simulink model "robot"  (R2019b)
settings: Solver=VariableStepAuto  StartTime=0.0  StopTime=45  RelTol=1e-3
values from neighbouring files (symbols this model uses):
  kf = 20    [workspace.mat]
  km = 0.4872    [workspace.mat]
  kp = 10    [workspace.mat]
  momemt_of_inertia = 0.0024    [workspace.mat]
  targets = [1  1; 2  1; -1  -1; -1  1; 0  0]    [workspace.mat]
  wheel_radius = 0.02    [workspace.mat]
  wheel_span = 0.1    [workspace.mat]
  winding_inductance = 0.0047    [workspace.mat]
  winding_resistance = 8.4929    [workspace.mat]
libraries: dspsigops x1, simulink x1
settings Model: Creator=Gudini  LastModifiedBy=Gudini

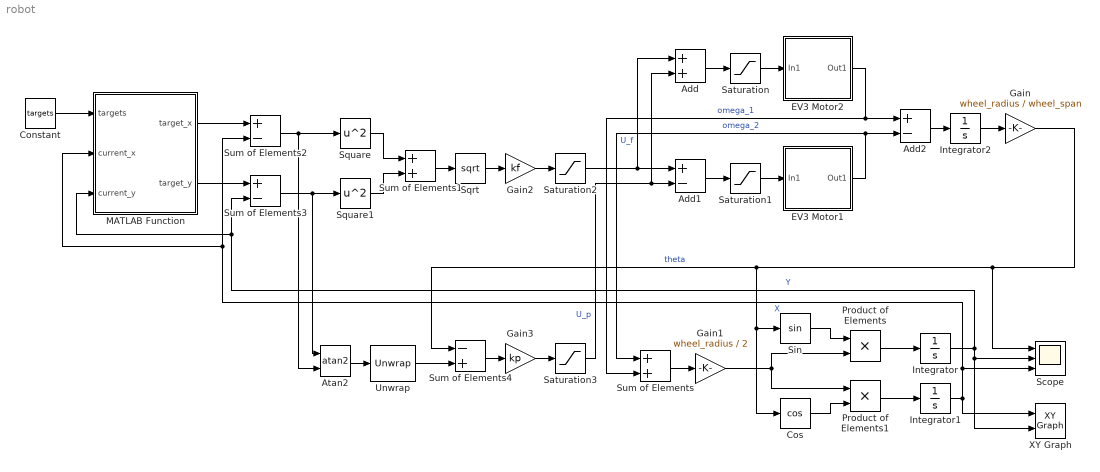
== system robot ==
  Add : Sum
  Add1 : Sum  Inputs=+-
  Add2 : Sum  Inputs=+-
  Atan2 : Trigonometry  Operator=atan2
  Constant : Constant  Value=targets  VectorParams1D=off
  Cos : Trigonometry  Operator=cos
  EV3 Motor1 : Subsystem
  EV3 Motor2 : Subsystem
  Gain : Gain  Gain=wheel_radius / wheel_span
  Gain1 : Gain  Gain=wheel_radius / 2
  Gain2 : Gain  Gain=kf
  Gain3 : Gain  Gain=kp
  Integrator : Integrator
  Integrator1 : Integrator
  Integrator2 : Integrator
  MATLAB Function : MATLAB Function  TreatAsAtomicUnit=on
  Product of Elements : Product
  Product of Elements1 : Product
  Saturation : Saturate  UpperLimit=7.6  LowerLimit=-7.6  ZeroCross=off
  Saturation1 : Saturate  UpperLimit=7.6  LowerLimit=-7.6  ZeroCross=off
  Saturation2 : Saturate  UpperLimit=7.6  LowerLimit=-7.6
  Saturation3 : Saturate  UpperLimit=7.6  LowerLimit=-7.6
  Scope : Scope  NumInputPorts=3
  Sin : Trigonometry
  Sqrt : Sqrt  SaturateOnIntegerOverflow=on
  Square : Math  Operator=square  SignedPower=off  SaturateOnIntegerOverflow=on
  Square1 : Math  Operator=square  SignedPower=off  SaturateOnIntegerOverflow=on
  Sum of Elements : Sum
  Sum of Elements1 : Sum
  Sum of Elements2 : Sum  Inputs=+-
  Sum of Elements3 : Sum  Inputs=+-
  Sum of Elements4 : Sum  Inputs=-+
  Unwrap : dspsigops/Unwrap  tol=pi  InputProcessing=Columns as channels (frame based)  running=off
  XY Graph : simulink/Sinks/XY Graph  xmin=-2  xmax=2  ymin=-2  ymax=2  st=-1
  wires:
  Add/1 -> Saturation/1
  Saturation/1 -> EV3 Motor2/1(In1)
  Saturation1/1 -> EV3 Motor1/1(In1)
  Add1/1 -> Saturation1/1
  Sin/1 -> Product of Elements/1
  Gain1/1 -> Product of Elements1/1, Product of Elements/2
  Cos/1 -> Product of Elements1/2
  Product of Elements/1 -> Integrator/1
  Product of Elements1/1 -> Integrator1/1
  Sum of Elements/1 -> Gain1/1
  EV3 Motor1/1(Out1) -> Sum of Elements/1, Add2/2  "omega_2"
  EV3 Motor2/1(Out1) -> Add2/1, Sum of Elements/2  "omega_1"
  Saturation2/1 -> Add/1, Add1/1  "U_f"
  Saturation3/1 -> Add/2, Add1/2  "U_p"
  Gain2/1 -> Saturation2/1
  Gain3/1 -> Saturation3/1
  Sqrt/1 -> Gain2/1
  Sum of Elements1/1 -> Sqrt/1
  Square1/1 -> Sum of Elements1/2
  Square/1 -> Sum of Elements1/1
  Sum of Elements3/1 -> Square1/1, Atan2/1
  Sum of Elements2/1 -> Square/1, Atan2/2
  MATLAB Function/2(target_y) -> Sum of Elements3/1
  MATLAB Function/1(target_x) -> Sum of Elements2/1
  Gain/1 -> Scope/1, Sum of Elements4/1, Cos/1, Sin/1  "theta"
  Integrator/1 -> XY Graph/2, Scope/2, MATLAB Function/3(current_y), Sum of Elements3/2  "Y"
  Integrator1/1 -> XY Graph/1, Sum of Elements2/2, MATLAB Function/2(current_x), Scope/3  "X"
  Sum of Elements4/1 -> Gain3/1
  Add2/1 -> Integrator2/1
  Integrator2/1 -> Gain/1
  Constant/1 -> MATLAB Function/1(targets)
  Unwrap/1 -> Sum of Elements4/2
  Atan2/1 -> Unwrap/1

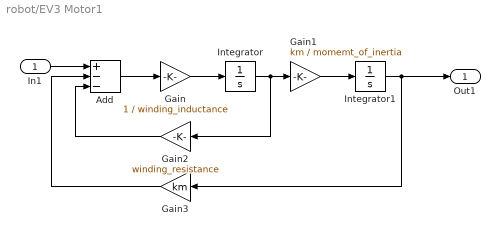
== system robot/EV3 Motor1 ==
  In1 : Inport
  Add : Sum  Inputs=+--
  Gain : Gain  Gain=1 / winding_inductance
  Gain1 : Gain  Gain=km / momemt_of_inertia
  Gain2 : Gain  Gain=winding_resistance
  Gain3 : Gain  Gain=km
  Integrator : Integrator
  Integrator1 : Integrator
  Out1 : Outport
  wires:
  Gain1/1 -> Integrator1/1
  In1/1 -> Add/1
  Integrator1/1 -> Out1/1, Gain3/1
  Integrator/1 -> Gain2/1, Gain1/1
  Gain/1 -> Integrator/1
  Gain2/1 -> Add/3
  Add/1 -> Gain/1
  Gain3/1 -> Add/2

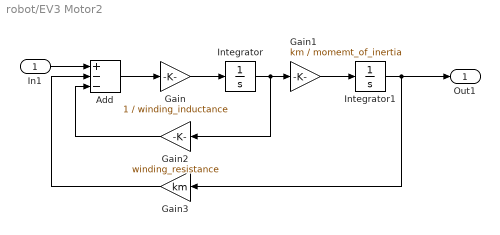
== system robot/EV3 Motor2 ==
  In1 : Inport
  Add : Sum  Inputs=+--
  Gain : Gain  Gain=1 / winding_inductance
  Gain1 : Gain  Gain=km / momemt_of_inertia
  Gain2 : Gain  Gain=winding_resistance
  Gain3 : Gain  Gain=km
  Integrator : Integrator
  Integrator1 : Integrator
  Out1 : Outport
  wires:
  Gain1/1 -> Integrator1/1
  In1/1 -> Add/1
  Integrator1/1 -> Out1/1, Gain3/1
  Integrator/1 -> Gain2/1, Gain1/1
  Gain/1 -> Integrator/1
  Gain2/1 -> Add/3
  Add/1 -> Gain/1
  Gain3/1 -> Add/2

== matlab function robot/MATLAB Function ==
  settings: updateMethod=DISCRETE  sampleTime=0.1
  data: targets input; target_x output; target_y output; current_x input; current_y input
function [target_x, target_y]= target_state(targets, current_x, current_y)
persistent state;
if isempty(state)
    state = 1;
end

target = targets(state, :);

if abs(current_x - target(1)) < 0.05 && abs(current_y - target(2)) < 0.05
    if state < size(targets, 1)
        state = state + 1;
    end
end
target = targets(state, :);
target_x = target(1);
target_y = target(2);
